simulink model "CloudLab_simulation"  (R2013b)
settings: Solver=ode3  StartTime=0.0  StopTime=10  RelTol=1e-3
values from neighbouring files (symbols this model uses):
  K = place(A,B,P)    [runParameters.m]
  K1 = 20    [runParameters.m]
  sigma002 = (rho0/rho7)*1    (= 0.0255139145777)    [runParameters.m]
  sigma01 = rho0/rho7    (= 0.0255139145777)    [runParameters.m]
  sigma102 = (rho1/rho7)*1    (= 0.245877856025)    [runParameters.m]
  sigma11 = rho1/rho7    (= 0.245877856025)    [runParameters.m]
  sigma202 = (rho2/rho7)*1    (= 0.0127569572888)    [runParameters.m]
  sigma21 = rho2/rho7    (= 0.0127569572888)    [runParameters.m]
  sigma302 = (rho3/rho7)*1    (= 0.029766233674)    [runParameters.m]
  sigma31 = rho3/rho7    (= 0.029766233674)    [runParameters.m]
  sigma402 = (rho4/rho7)*1    (= 0.01826)    [runParameters.m]
  sigma502 = (rho5/rho7)*1    (= 0.00108724067803)    [runParameters.m]
  sigma602 = (rho6/rho7)*1    (= 1.56432188754)    [runParameters.m]
  sigma61 = rho6/rho7    (= 1.56432188754)    [runParameters.m]
  vs1 = -sigma01*sigma21/sigma31    (= -0.010934534819)    [runParameters.m]
  vs2 = sigma01*sigma51/sigma31    (= 0.000931920581165)    [runParameters.m]
  vs3 = -sigma01*sigma61/sigma31    (= -1.34084733218)    [runParameters.m]
  vs4 = 2*sigma21    (= 0.0255139145777)    [runParameters.m]
  vs5 = sigma41    (= 0.01826)    [runParameters.m]
  vs6 = sigma01    (= 0.0255139145777)    [runParameters.m]
settings Model: Creator=vss  LastModifiedBy=Pikachu
settings SolverCC: ZeroCrossAlgorithm=Adaptive
settings DataIOCC: SignalLoggingSaveFormat=ModelDataLogs
settings DebuggingCC: MultiTaskDSMMsg=warning  MultiTaskCondExecSysMsg=none  FrameProcessingCompatibilityMsg=error  StateNameClashWarn=warning
settings RTWCC: IncludeERTFirstTime=on
settings GRTTargetCC: CodeReplacementLibrary=C89/C90 (ANSI)
settings ConfigurationSet: Description=SimMechanics 2G

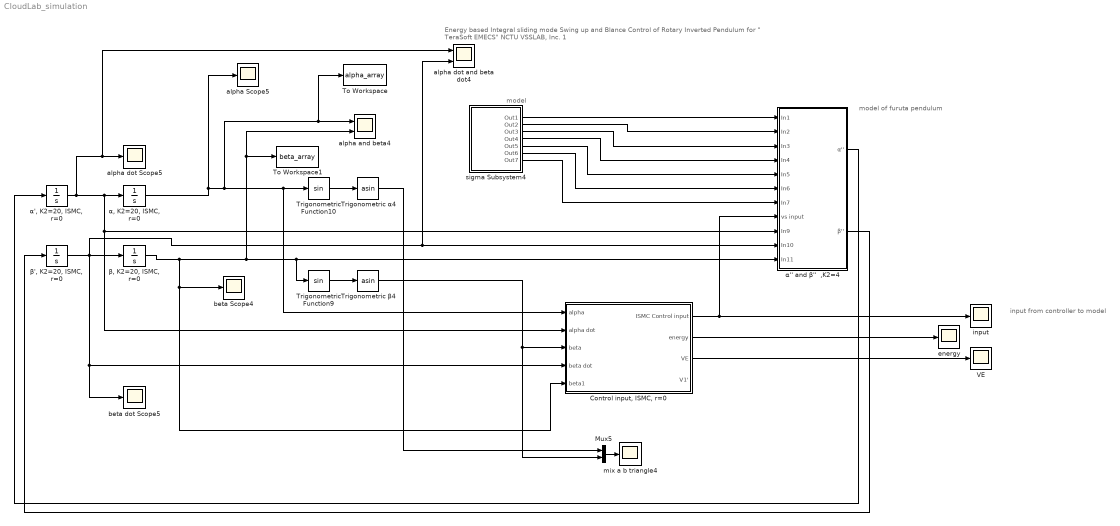
== system CloudLab_simulation ==
  note: input from controller to model
  note: model of furuta pendulum
  note: model
  note: Energy based Integral sliding mode Swing up and Blance Control of Rotary Inverted Pendulum for " TeraSoft EMECS"
      |                                                              NCTU VSSLAB, Inc. 1
  " Control input, ISMC, r=0" : Subsystem
  Mux5 : Mux  Inputs=2
  To Workspace : ToWorkspace  VariableName=alpha_array  SampleTime=0.04
  To Workspace1 : ToWorkspace  VariableName=beta_array  SampleTime=0.04
  Trigonometric Function10 : Trigonometry
  Trigonometric Function9 : Trigonometry
  Trigonometric α4 : Trigonometry  Operator=asin
  Trigonometric β4 : Trigonometry  Operator=asin
  VE : Scope
      settings: ShowLegends=on  TimeRange=1  YMin=6.28316  YMax=6.28319
  alpha Scope5 : Scope
      settings: TimeRange=10  YMin=-3.5  YMax=6.5  SaveName=ScopeData42
  alpha and beta4 : Scope  NumInputPorts=2
      settings: ShowLegends=on  TimeRange=10  YMin=-3.5~-5  YMax=6.5~5  SaveName=ScopeData43
  alpha dot Scope5 : Scope
      settings: YMin=-10  YMax=10  SaveName=ScopeData44
  alpha dot and beta dot4 : Scope  NumInputPorts=2
      settings: ShowLegends=on  TimeRange=10  YMin=-3.5~-5  YMax=6.5~5  SaveName=ScopeData45
  beta Scope4 : Scope
      settings: TimeRange=1  YMin=0.25  YMax=3.25  SaveName=ScopeData46
  beta dot Scope5 : Scope
      settings: TimeRange=6  YMin=-2.75  YMax=0.5  SaveName=ScopeData47
  energy : Scope
      settings: ShowLegends=on  TimeRange=1  YMin=6.28316  YMax=6.28319
  input : Scope
      settings: ShowLegends=on  TimeRange=1  YMin=6.28316  YMax=6.28319  SaveName=ScopeData3
  mix a b triangle4 : Scope
      settings: ShowLegends=on  TimeRange=1  YMin=6.28316  YMax=6.28319  SaveName=ScopeData48
  sigma Subsystem4 : Subsystem
  α'' and β''  ,K2=4 : Subsystem
  "α', K2=20, ISMC, r=0" : Integrator
  "α, K2=20, ISMC, r=0" : Integrator
  "β', K2=20, ISMC, r=0" : Integrator
  "β, K2=20, ISMC, r=0" : Integrator  InitialCondition=pi  UpperSaturationLimit=7  LowerSaturationLimit=0
  wires:
  "α', K2=20, ISMC, r=0"/1 -> alpha dot and beta dot4/1, alpha dot Scope5/1, " Control input, ISMC, r=0"/2(alpha dot), α'' and β''  ,K2=4/9(In9), "α, K2=20, ISMC, r=0"/1
  α'' and β''  ,K2=4/2(β'') -> "β', K2=20, ISMC, r=0"/1
  "β, K2=20, ISMC, r=0"/1 -> " Control input, ISMC, r=0"/5(beta1), beta Scope4/1, To Workspace1/1, alpha and beta4/2, α'' and β''  ,K2=4/11(In11), Trigonometric Function9/1
  Trigonometric Function9/1 -> Trigonometric β4/1
  Trigonometric β4/1 -> Mux5/2, " Control input, ISMC, r=0"/3(beta)
  α'' and β''  ,K2=4/1(α'') -> "α', K2=20, ISMC, r=0"/1
  sigma Subsystem4/1(Out1) -> α'' and β''  ,K2=4/1(In1)
  sigma Subsystem4/2(Out2) -> α'' and β''  ,K2=4/2(In2)
  sigma Subsystem4/3(Out3) -> α'' and β''  ,K2=4/3(In3)
  sigma Subsystem4/4(Out4) -> α'' and β''  ,K2=4/4(In4)
  sigma Subsystem4/5(Out5) -> α'' and β''  ,K2=4/5(In5)
  sigma Subsystem4/6(Out6) -> α'' and β''  ,K2=4/6(In6)
  sigma Subsystem4/7(Out7) -> α'' and β''  ,K2=4/7(In7)
  Trigonometric Function10/1 -> Trigonometric α4/1
  Trigonometric α4/1 -> Mux5/1
  Mux5/1 -> mix a b triangle4/1
  "β', K2=20, ISMC, r=0"/1 -> beta dot Scope5/1, " Control input, ISMC, r=0"/4(beta dot), "β, K2=20, ISMC, r=0"/1, alpha dot and beta dot4/2, α'' and β''  ,K2=4/10(In10)
  " Control input, ISMC, r=0"/2(energy) -> energy/1
  " Control input, ISMC, r=0"/3(" VE") -> VE/1
  " Control input, ISMC, r=0"/1(ISMC Control input) -> α'' and β''  ,K2=4/8(vs input), input/1
  "α, K2=20, ISMC, r=0"/1 -> alpha Scope5/1, To Workspace/1, alpha and beta4/1, " Control input, ISMC, r=0"/1(alpha), Trigonometric Function10/1

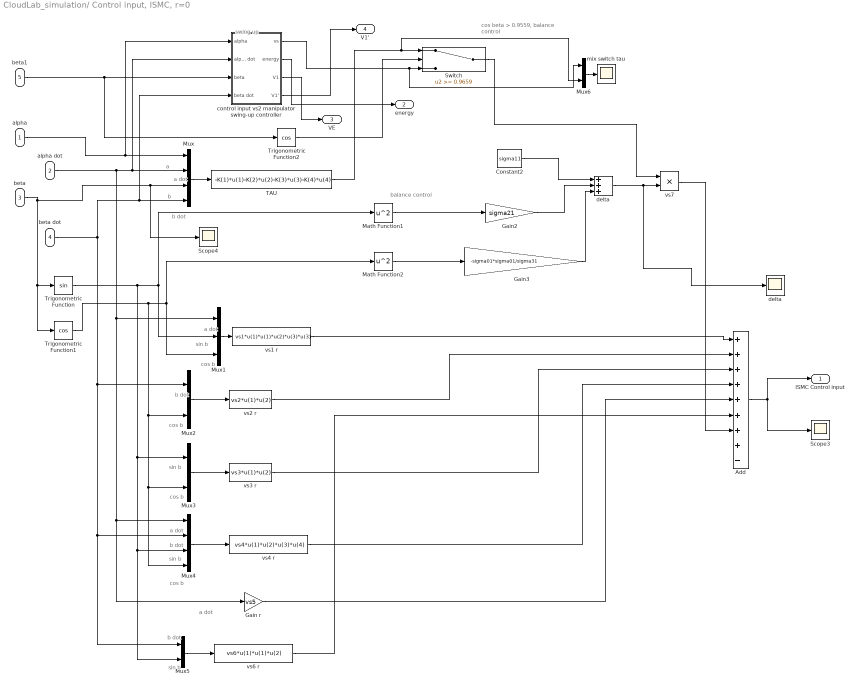
== system CloudLab_simulation/ Control input, ISMC, r=0 ==
  note: cos beta > 0.9559, balance control
  note: swing up
  note: balance control
  note: sin b
  note: b dot
  note: a dot
  note: cos b
  note: sin b
  note: b dot
  note: a dot
  note: cos b
  note: sin b
  note: cos b
  note: b dot
  note: cos b
  note: sin b
  note: a dot
  note: b dot
  note: b
  note: a dot
  note: a
  alpha : Inport
  alpha dot : Inport  Port=2
  beta : Inport  Port=3
  beta dot : Inport  Port=4
  beta1 : Inport  Port=5
  Add : Sum  Inputs=++++++++-
  Constant2 : Constant  Value=sigma11
  Gain r : Gain  Gain=vs5
  Gain2 : Gain  Gain=sigma21
  Gain3 : Gain  Gain=-sigma01*sigma01/sigma31
  Math Function1 : Math  Operator=square  SaturateOnIntegerOverflow=on
  Math Function2 : Math  Operator=square  SaturateOnIntegerOverflow=on
  Mux : Mux
  Mux1 : Mux  Inputs=3
  Mux{2..3,5..6} (4 alike) : Mux  Inputs=2
  Mux4 : Mux
  Scope3 : Scope
      settings: YMin=-10  YMax=10  SaveName=ScopeData4
  Scope4 : Scope
      settings: YMin=-10  YMax=10  SaveName=ScopeData12
  Switch : Switch  Threshold=0.9659
  TAU : Fcn  Expr=-K(1)*u(1)-K(2)*u(2)-K(3)*u(3)-K(4)*u(4)
  Trigonometric Function : Trigonometry
  Trigonometric Function1 : Trigonometry  Operator=cos
  Trigonometric Function2 : Trigonometry  Operator=cos
  control input vs2 manipulator swing-up controller : Subsystem
  delta : Sum  Inputs=+++
  "delta " : Scope
      settings: YMin=-10  YMax=10  SaveName=ScopeData8
  mix switch tau : Scope
      settings: ShowLegends=on  TimeRange=1  YMin=6.28316  YMax=6.28319  SaveName=ScopeData14
  vs1 r : Fcn  Expr=vs1*u(1)*u(1)*u(2)*u(3)*u(3)
  vs2 r : Fcn  Expr=vs2*u(1)*u(2)
  vs3 r : Fcn  Expr=vs3*u(1)*u(2)
  "vs4 r " : Fcn  Expr=vs4*u(1)*u(2)*u(3)*u(4)
  "vs6 r " : Fcn  Expr=vs6*u(1)*u(1)*u(2)
  vs7 : Product
  ISMC Control input : Outport
  energy : Outport  Port=2
  " VE" : Outport  Port=3
  "V1' " : Outport  Port=4
  wires:
  Mux/1 -> TAU/1
  alpha/1 -> control input vs2 manipulator swing-up controller/1(alpha), Mux/1
  beta/1 -> Trigonometric Function/1, Trigonometric Function1/1, Scope4/1, Mux/3
  Trigonometric Function/1 -> Mux5/2, Mux4/3, Mux3/1, Math Function1/1, Mux1/2
  Trigonometric Function1/1 -> Mux2/2, Mux3/2, Mux4/4, Math Function2/1, Mux1/3
  Mux1/1 -> vs1 r/1
  Mux2/1 -> vs2 r/1
  Mux3/1 -> vs3 r/1
  Mux4/1 -> "vs4 r "/1
  Add/1 -> Scope3/1, ISMC Control input/1
  vs1 r/1 -> Add/1
  vs2 r/1 -> Add/2
  vs3 r/1 -> Add/3
  "vs4 r "/1 -> Add/4
  Gain r/1 -> Add/5
  Constant2/1 -> delta/1
  Math Function1/1 -> Gain2/1
  Gain2/1 -> delta/2
  Gain3/1 -> delta/3
  Math Function2/1 -> Gain3/1
  delta/1 -> "delta "/1, vs7/2
  vs7/1 -> Add/7
  alpha dot/1 -> control input vs2 manipulator swing-up controller/2(alpha dot), Mux/2, Mux4/1, Gain r/1, Mux1/1
  beta dot/1 -> Mux4/2, Mux5/1, Mux2/1, control input vs2 manipulator swing-up controller/4(beta dot), Mux/4
  Mux5/1 -> "vs6 r "/1
  "vs6 r "/1 -> Add/6
  Switch/1 -> vs7/1
  beta1/1 -> Trigonometric Function2/1, control input vs2 manipulator swing-up controller/3(beta)
  TAU/1 -> Mux6/2, Switch/1
  control input vs2 manipulator swing-up controller/1(vs) -> Mux6/1, Switch/3
  Mux6/1 -> mix switch tau/1
  control input vs2 manipulator swing-up controller/4("V1' ") -> "V1' "/1
  control input vs2 manipulator swing-up controller/3(" V1") -> " VE"/1
  control input vs2 manipulator swing-up controller/2(energy) -> energy/1
  Trigonometric Function2/1 -> Switch/2

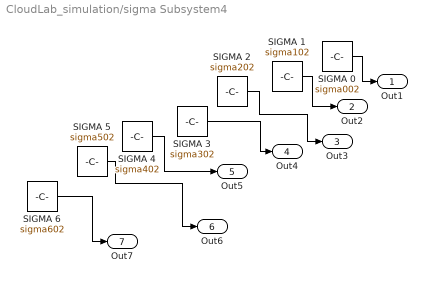
== system CloudLab_simulation/sigma Subsystem4 ==
  SIGMA 0 : Constant  Value=sigma002
  SIGMA 1 : Constant  Value=sigma102
  SIGMA 2 : Constant  Value=sigma202
  SIGMA 3 : Constant  Value=sigma302
  SIGMA 4 : Constant  Value=sigma402
  SIGMA 5 : Constant  Value=sigma502
  SIGMA 6 : Constant  Value=sigma602
  Out1 : Outport
  Out2 : Outport  Port=2
  Out3 : Outport  Port=3
  Out4 : Outport  Port=4
  Out5 : Outport  Port=5
  Out6 : Outport  Port=6
  Out7 : Outport  Port=7
  wires:
  SIGMA 0/1 -> Out1/1
  SIGMA 1/1 -> Out2/1
  SIGMA 2/1 -> Out3/1
  SIGMA 3/1 -> Out4/1
  SIGMA 4/1 -> Out5/1
  SIGMA 5/1 -> Out6/1
  SIGMA 6/1 -> Out7/1

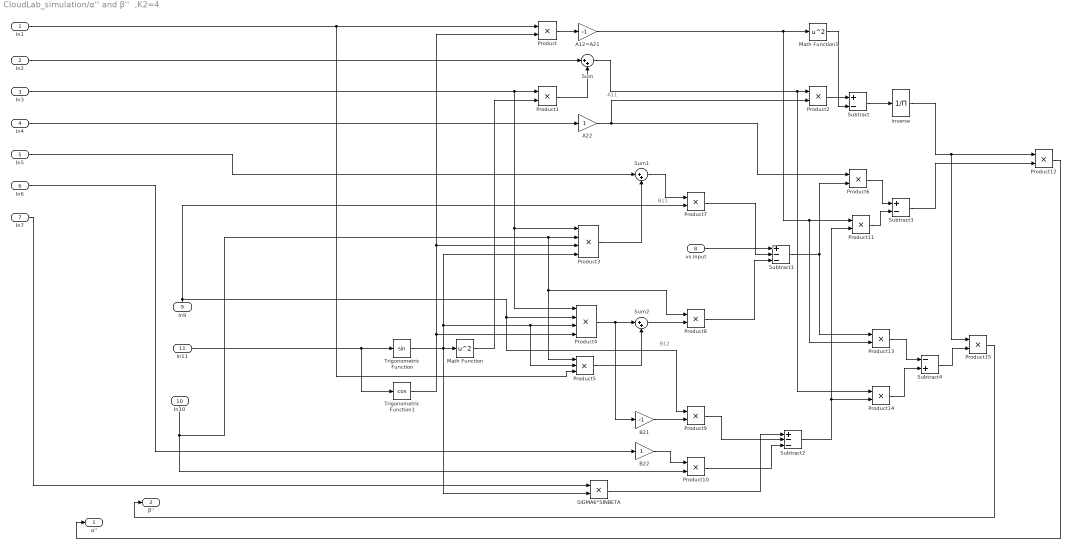
== system CloudLab_simulation/α'' and β''  ,K2=4 ==
  note: vs
  note: B12
  note: B11
  note: A11
  In1 : Inport
  In2 : Inport  Port=2
  In3 : Inport  Port=3
  In4 : Inport  Port=4
  In5 : Inport  Port=5
  In6 : Inport  Port=6
  In7 : Inport  Port=7
  vs input : Inport  Port=8
  In9 : Inport  Port=9
  In10 : Inport  Port=10
  In11 : Inport  Port=11
  A12=A21 : Gain  Gain=-1
  A22 : Gain
  B21 : Gain  Gain=-1
  B22 : Gain
  Math Function : Math  Operator=square  SaturateOnIntegerOverflow=on
  Math Function1 : Math  Operator=square  SaturateOnIntegerOverflow=on
  Product{,1..2,6..15} (13 alike) : Product
  Product3 : Product  Inputs=4
  Product4 : Product  Inputs=4
  Product5 : Product  Inputs=3
  SIGMA6*SINBETA : Product
  Subtract : Sum  Inputs=+-
  Subtract1 : Sum  Inputs=+--
  Subtract2 : Sum  Inputs=+--
  Subtract3 : Sum  Inputs=+-
  Subtract4 : Sum  Inputs=-+
  Sum : Sum  Inputs=|++
  Sum1 : Sum  Inputs=|++
  Sum2 : Sum  Inputs=|++
  Trigonometric Function : Trigonometry
  Trigonometric Function1 : Trigonometry  Operator=cos
  inverse : Product  Inputs=/  SaturateOnIntegerOverflow=on  RndMeth=Zero  InputSameDT=on  OutDataTypeStr=Inherit: Same as first input
  α'' : Outport
  β'' : Outport  Port=2
  wires:
  Product8/1 -> Subtract1/3
  B22/1 -> Product10/1
  Product9/1 -> Subtract2/2
  Product10/1 -> Subtract2/3
  Subtract1/1 -> Product6/2, Product13/1
  Product6/1 -> Subtract3/1
  Product11/1 -> Subtract3/2
  Subtract2/1 -> Product14/2, Product11/2
  inverse/1 -> Product15/1, Product12/1
  Subtract3/1 -> Product12/2
  Product12/1 -> α''/1
  Product13/1 -> Subtract4/1
  Product14/1 -> Subtract4/2
  Subtract4/1 -> Product15/2
  Product15/1 -> β''/1
  B21/1 -> Product9/2
  In11/1 -> Trigonometric Function1/1, Trigonometric Function/1
  vs input/1 -> Subtract1/1
  In10/1 -> Product10/2, Product8/1, Product5/1, Product3/2
  In9/1 -> Product9/1, Product4/2, Product7/2
  Math Function1/1 -> Subtract/2
  Trigonometric Function/1 -> SIGMA6*SINBETA/2, Product5/2, Product4/3, Product3/4, Math Function/1
  Math Function/1 -> Product1/2
  In3/1 -> Product4/1, Product3/1, Product1/1
  Product1/1 -> Sum/2
  A12=A21/1 -> Product13/2, Product11/1, Math Function1/1
  In7/1 -> SIGMA6*SINBETA/1
  In1/1 -> Product/1, Product5/3
  In2/1 -> Sum/1
  Trigonometric Function1/1 -> Product4/4, Product3/3, Product/2
  Product/1 -> A12=A21/1
  In4/1 -> A22/1
  Sum/1 -> Product14/1, Product2/1
  A22/1 -> Product6/1, Product2/2
  Product2/1 -> Subtract/1
  Product3/1 -> Sum1/2
  Subtract/1 -> inverse/1
  In5/1 -> Sum1/1
  Product4/1 -> B21/1, Sum2/1
  Product5/1 -> Sum2/2
  In6/1 -> B22/1
  Sum1/1 -> Product7/1
  Sum2/1 -> Product8/2
  SIGMA6*SINBETA/1 -> Subtract2/1
  Product7/1 -> Subtract1/2

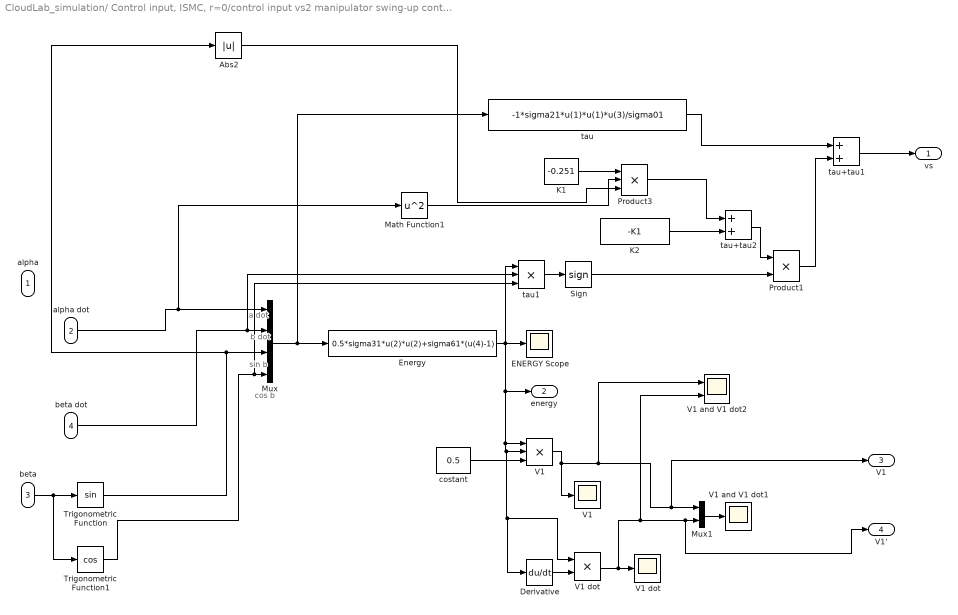
== system CloudLab_simulation/ Control input, ISMC, r=0/control input vs2 manipulator swing-up controller ==
  note: cos b
  note: sin b
  note: b dot
  note: a dot
  alpha : Inport
  alpha dot : Inport  Port=2
  beta : Inport  Port=3
  beta dot : Inport  Port=4
  Abs2 : Abs  SaturateOnIntegerOverflow=on
  Derivative : Derivative
  ENERGY Scope : Scope
      settings: YMin=-10  YMax=10  SaveName=ScopeData27
  "Energy " : Fcn  Expr=0.5*sigma31*u(2)*u(2)+sigma61*(u(4)-1)
  K1 : Constant  Value=-0.251
  K2 : Constant  Value=-K1
  Math Function1 : Math  Operator=square  SaturateOnIntegerOverflow=on
  Mux : Mux
  Mux1 : Mux  Inputs=2
  Product1 : Product
  Product3 : Product  Inputs=3
  Sign : Signum  ZeroCross=off
  Trigonometric Function : Trigonometry
  Trigonometric Function1 : Trigonometry  Operator=cos
  V1 : Scope
      settings: YMin=-10  YMax=10  SaveName=ScopeData17
  "V1 " : Product  Inputs=3
  V1 and V1 dot1 : Scope
      settings: ShowLegends=on  YMin=-10  YMax=10  SaveName=ScopeData19
  V1 and V1 dot2 : Scope  NumInputPorts=2
      settings: ShowLegends=on  YMin=-5~-5  YMax=5~5  SaveName=ScopeData10
  V1 dot : Scope
      settings: YMin=-10  YMax=10  SaveName=ScopeData18
  "V1 dot " : Product
  costant : Constant  Value=0.5
  tau : Fcn  Expr=-1*sigma21*u(1)*u(1)*u(3)/sigma01
  tau+tau1 : Sum
  tau+tau2 : Sum
  tau1 : Product  Inputs=3
  vs : Outport
  energy : Outport  Port=2
  " V1" : Outport  Port=3
  "V1' " : Outport  Port=4
  wires:
  beta/1 -> Trigonometric Function/1, Trigonometric Function1/1
  Trigonometric Function/1 -> Mux/3, Abs2/1
  Trigonometric Function1/1 -> tau1/3, Mux/4
  beta dot/1 -> tau1/2, Mux/2
  Mux/1 -> tau/1, "Energy "/1
  "Energy "/1 -> "V1 "/1, Derivative/1, "V1 dot "/1, "V1 "/2, energy/1, ENERGY Scope/1, tau1/1
  tau/1 -> tau+tau1/1
  tau+tau1/1 -> vs/1
  tau1/1 -> Sign/1
  costant/1 -> "V1 "/3
  "V1 "/1 -> V1 and V1 dot2/1, " V1"/1, Mux1/1, V1/1
  Derivative/1 -> "V1 dot "/2
  "V1 dot "/1 -> V1 and V1 dot2/2, "V1' "/1, Mux1/2, V1 dot/1
  Mux1/1 -> V1 and V1 dot1/1
  K1/1 -> Product3/1
  alpha dot/1 -> Math Function1/1, Mux/1
  Math Function1/1 -> Product3/2
  Product3/1 -> tau+tau2/1
  K2/1 -> tau+tau2/2
  Sign/1 -> Product1/2
  tau+tau2/1 -> Product1/1
  Product1/1 -> tau+tau1/2
  Abs2/1 -> Product3/3
